simulink model "system_blocks"  (R2019b)
settings: Solver=ode4  StartTime=t_start  StopTime=t_stop  FixedStep=t_step  RelTol=1e-3
libraries: mpclib x3
settings Model: Creator=Vish  LastModifiedBy=Vish

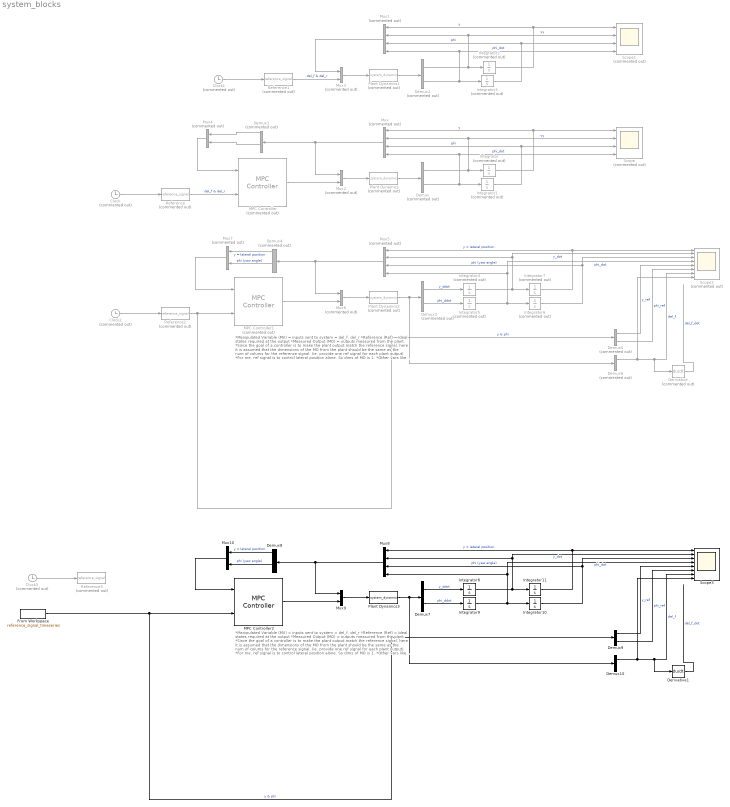
== system system_blocks ==
  note: *Manipulated Variable (MV) = inputs sent to system = del_f, del_r
      | *Reference (Ref) = Ideal states required at the output
      | *Measured Output (MO) = outputs measured from the plant.
      |
      | *Since the goal of a controller is to make the plant output match
      | the reference signal, here it is assumed that the dimensions of
      | the MO from the plant should be the same as the num of colums
      | for the reference signal. (ie. provide one ref signal for each plant output)
      | *For me, ref signal is to control lateral position alone. So dims of MO is 1.
      | *Other vars like yaw angle/yaw rate is only for analysis purpose to see if
      | with dual steer, the plant requires less control effort for high yaw rate/high
      | lateral position...which as per eqns it should since an extra addition term
      | corsp to del_r is added to the y_ddot and phi_ddot eqns.
      |
      | ** Procedure:
      | *1. Add MPC block.
      | *2. Double click MPC block and Uncheck Measured Disturbance (MD)
      | *2.1 Connect the block to proposed input ref signal block and input of plant. This
      | will allow it to auto-generate potential MO and MV signals and extract dimension
      | of those signals from there.
      | *3. Double click on MPC block and click Design button next to "Controller" textbox
      | *4. Select correct input and output signal paths from simulink block in case block
      | had picked wrong signals or you want a particulr demuxed signal at output. To do
      | so, at the bottom, click on "Select Signals" next to "Block Path", select line in model,
      | choose "add".
      | *5. Now set MV and MO dimensions for the corresponding signal paths/ports by
      | clicking "Change I/O Sizes" at the top right.
  note: *Manipulated Variable (MV) = inputs sent to system = del_f, del_r
      | *Reference (Ref) = Ideal states required at the output
      | *Measured Output (MO) = outputs measured from the plant.
      |
      | *Since the goal of a controller is to make the plant output match
      | the reference signal, here it is assumed that the dimensions of
      | the MO from the plant should be the same as the num of colums
      | for the reference signal. (ie. provide one ref signal for each plant output)
      | *For me, ref signal is to control lateral position alone. So dims of MO is 1.
      | *Other vars like yaw angle/yaw rate is only for analysis purpose to see if
      | with dual steer, the plant requires less control effort for high yaw rate/high
      | lateral position...which as per eqns it should since an extra addition term
      | corsp to del_r is added to the y_ddot and phi_ddot eqns.
      |
      | ** Procedure:
      | *1. Add MPC block.
      | *2. Double click MPC block and Uncheck Measured Disturbance (MD)
      | *2.1 Connect the block to proposed input ref signal block and input of plant. This
      | will allow it to auto-generate potential MO and MV signals and extract dimension
      | of those signals from there.
      | *3. Double click on MPC block and click Design button next to "Controller" textbox
      | *4. Select correct input and output signal paths from simulink block in case block
      | had picked wrong signals or you want a particulr demuxed signal at output. To do
      | so, at the bottom, click on "Select Signals" next to "Block Path", select line in model,
      | choose "add".
      | *5. Now set MV and MO dimensions for the corresponding signal paths/ports by
      | clicking "Change I/O Sizes" at the top right.
  Clock{,1..3} (4 alike) : Clock  Commented=on
  Demux{,2..3,5..6} (5 alike) : Demux  Commented=on  Outputs=2
  Demux1 : Demux  Commented=on
  Demux10 : Demux  Outputs=2
  Demux4 : Demux  Commented=on
  Demux7 : Demux  Outputs=2
  Demux8 : Demux
  Demux9 : Demux  Outputs=2
  Derivative : Derivative  Commented=on
  Derivative1 : Derivative
  From Workspace : FromWorkspace  VariableName=reference_signal_timeseries  SampleTime=0
  Integrator{,1..7} (8 alike) : Integrator  Commented=on
  Integrator{8..11} (4 alike) : Integrator
  MPC Controller : mpclib/MPC Controller  Commented=on  SCDEnableBlockLinearizationSpecification=on  is_multiple=0  enable_value=0  return_u0=off  updateMPCinCallerWorkspace=on  md_inport=off  mv_inport=off  uref_inport=off  return_cost=off  return_mvseq=off  return_qpstatus=off  return_xseq=off  return_state=off  return_ovseq=off  state_inport=off  umin_inport=off  umax_inport=off  ymin_inport=off  ymax_inport=off  cc_inport=off  ywt_inport=off  uwt_inport=off  duwt_inport=off  rhoeps_inport=off  pm_inport=off  MaximumP=10  HorizonChoice=FixedHorizon  n_ts=0.1  n_p=10  n_mv=2  n_md=1  n_ud=0  n_mo=2  n_uo=0  BlockDataType=double  SampleTimeInherited=off  switch_inport=off
  MPC Controller1 : mpclib/MPC Controller  Commented=on  SCDEnableBlockLinearizationSpecification=on  mpcobj=mpc2  is_multiple=0  enable_value=0  return_u0=off  updateMPCinCallerWorkspace=on  md_inport=off  mv_inport=off  uref_inport=off  return_cost=off  return_mvseq=off  return_qpstatus=off  return_xseq=off  return_state=off  return_ovseq=off  state_inport=off  umin_inport=off  umax_inport=off  ymin_inport=off  ymax_inport=off  cc_inport=off  ywt_inport=off  uwt_inport=off  duwt_inport=off  rhoeps_inport=off  pm_inport=off  MaximumP=10  HorizonChoice=FixedHorizon  n_ts=0.1  n_p=10  n_mv=2  n_md=0  n_ud=0  n_mo=2  n_uo=0  BlockDataType=double  SampleTimeInherited=off  switch_inport=off
  MPC Controller2 : mpclib/MPC Controller  SCDEnableBlockLinearizationSpecification=on  mpcobj=mpc1  is_multiple=0  enable_value=0  return_u0=off  updateMPCinCallerWorkspace=on  md_inport=off  mv_inport=off  uref_inport=off  return_cost=off  return_mvseq=off  return_qpstatus=off  return_xseq=off  return_state=off  return_ovseq=off  state_inport=off  umin_inport=off  umax_inport=off  ymin_inport=off  ymax_inport=off  cc_inport=off  ywt_inport=off  uwt_inport=off  duwt_inport=off  rhoeps_inport=off  pm_inport=off  MaximumP=10  HorizonChoice=FixedHorizon  n_ts=0.1  n_p=10  n_mv=2  n_md=0  n_ud=0  n_mo=2  n_uo=0  BlockDataType=double  SampleTimeInherited=off  switch_inport=off
  Mux : Mux  Commented=on
  Mux1 : Mux  Commented=on
  Mux10 : Mux  Inputs=2
  Mux{2..4,6..7} (5 alike) : Mux  Commented=on  Inputs=2
  Mux5 : Mux  Commented=on
  Mux8 : Mux
  Mux9 : Mux  Inputs=2
  Plant Dynamics : MATLABFcn  Commented=on  MATLABFcn=system_dynamics  OutputDimensions=2
  Plant Dynamics1 : MATLABFcn  Commented=on  MATLABFcn=system_dynamics  OutputDimensions=2
  Plant Dynamics2 : MATLABFcn  Commented=on  MATLABFcn=system_dynamics  OutputDimensions=2
  Plant Dynamics3 : MATLABFcn  MATLABFcn=system_dynamics  OutputDimensions=2
  Reference{,1..3} (4 alike) : MATLABFcn  Commented=on  MATLABFcn=reference_signal  OutputDimensions=2
  Scope : Scope  Commented=on  NumInputPorts=4
  Scope1 : Scope  Commented=on  NumInputPorts=4
  Scope2 : Scope  Commented=on  NumInputPorts=8
  Scope3 : Scope  NumInputPorts=8
  wires:
  Plant Dynamics/1 -> Demux/1
  Demux/1 -> Mux/2, Scope/2, Integrator/1  "vy"
  Demux/2 -> Mux/4, Scope/4, Integrator1/1  "phi_dot"
  Integrator/1 -> Mux/1, Scope/1  "y"
  Integrator1/1 -> Mux/3, Scope/3  "phi"
  Mux2/1 -> Plant Dynamics/1
  Mux/1 -> Demux1/1, Mux2/1
  Demux2/2 -> Mux1/4, Scope1/4, Integrator3/1  "phi_dot"
  Plant Dynamics1/1 -> Demux2/1
  Integrator3/1 -> Mux1/3, Scope1/3  "phi"
  Demux2/1 -> Mux1/2, Scope1/2, Integrator2/1  "vy"
  Reference1/1 -> Mux3/2  "del_f & del_r"
  Mux3/1 -> Plant Dynamics1/1
  Integrator2/1 -> Mux1/1, Scope1/1  "y"
  Mux1/1 -> Mux3/1
  Clock1/1 -> Reference1/1
  Reference/1 -> MPC Controller/2  "del_f & del_r"
  Clock/1 -> Reference/1
  MPC Controller/1 -> Mux2/2
  Demux1/1 -> Mux4/1
  Demux1/3 -> Mux4/2
  Mux4/1 -> MPC Controller/1
  Demux3/2 -> Integrator5/1  "phi_ddot"
  Plant Dynamics2/1 -> Demux6/1, Demux3/1
  Integrator5/1 -> Scope2/4, Mux5/4, Integrator6/1  "phi_dot"
  Demux3/1 -> Integrator4/1  "y_ddot"
  Mux6/1 -> Plant Dynamics2/1
  Clock2/1 -> Reference2/1
  Mux5/1 -> Demux4/1, Mux6/1
  Reference2/1 -> MPC Controller1/2, Demux5/1  "y & phi"
  MPC Controller1/1 -> Mux6/2
  Integrator4/1 -> Scope2/2, Mux5/2, Integrator7/1  "y_dot"
  Integrator6/1 -> Mux5/3, Scope2/3  "phi (yaw angle)"
  Integrator7/1 -> Mux5/1, Scope2/1  "y = lateral position"
  Mux7/1 -> MPC Controller1/1
  Demux4/1 -> Mux7/1  "y = lateral position"
  Demux4/3 -> Mux7/2  "phi (yaw angle)"
  Demux5/1 -> Scope2/5  "y_ref"
  Demux5/2 -> Scope2/6  "phi_ref"
  Demux6/1 -> Scope2/8, Derivative/1, Scope2/7  "del_f"
  Derivative/1 -> ?  "del_f_dot"
  Demux10/1 -> Scope3/8, Derivative1/1, Scope3/7  "del_f"
  Integrator11/1 -> Mux8/1, Scope3/1  "y = lateral position"
  Mux10/1 -> MPC Controller2/1
  From Workspace/1 -> Demux9/1, MPC Controller2/2  "y & phi"
  Integrator10/1 -> Mux8/3, Scope3/3  "phi (yaw angle)"
  Demux7/1 -> Integrator8/1  "y_ddot"
  Demux8/1 -> Mux10/1  "y = lateral position"
  MPC Controller2/1 -> Mux9/2
  Mux9/1 -> Plant Dynamics3/1
  Demux7/2 -> Integrator9/1  "phi_ddot"
  Plant Dynamics3/1 -> Demux10/1, Demux7/1
  Demux9/2 -> Scope3/6  "phi_ref"
  Mux8/1 -> Demux8/1, Mux9/1
  Derivative1/1 -> ?  "del_f_dot"
  Integrator8/1 -> Scope3/2, Mux8/2, Integrator11/1  "y_dot"
  Integrator9/1 -> Scope3/4, Mux8/4, Integrator10/1  "phi_dot"
  Demux9/1 -> Scope3/5  "y_ref"
  Demux8/3 -> Mux10/2  "phi (yaw angle)"
  Clock3/1 -> Reference3/1
